simulink model "T_vs_pos_host"  (R2021b)
settings: Solver=ode1  StartTime=0.0  StopTime=inf  FixedStep=1e-3  RelTol=1e-3
libraries: slrealtimeutilitieslib x1, slrealtimeiplib x1
settings Model: Creator=tcraddoc  LastModifiedBy=wasynczu
settings SolverCC: AlgebraicLoopSolver=TrustRegion
settings DataIOCC: ReturnWorkspaceOutputs=off
settings DebuggingCC: SFMachineParentedDataDiag=warning  ArithmeticOperatorsInVariantConditions=warning
settings SFSimCC: SimUseLocalCustomCode=off  CustomCodeUndefinedFunction=UseInterfaceOnly
settings RTWCC: RTWUseLocalCustomCode=off
settings CodeAppCC: StateflowObjectComments=on

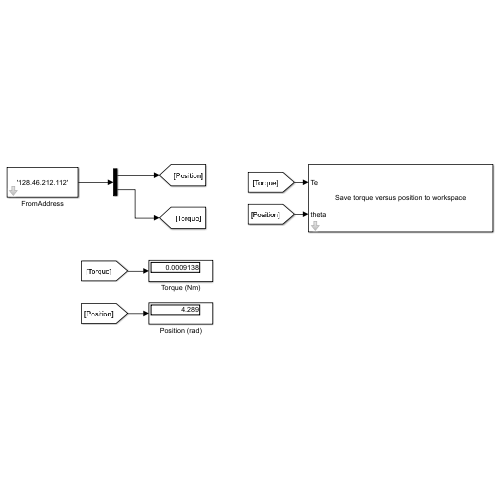
[thumbnail: Simulink's stored preview of the top-level diagram]
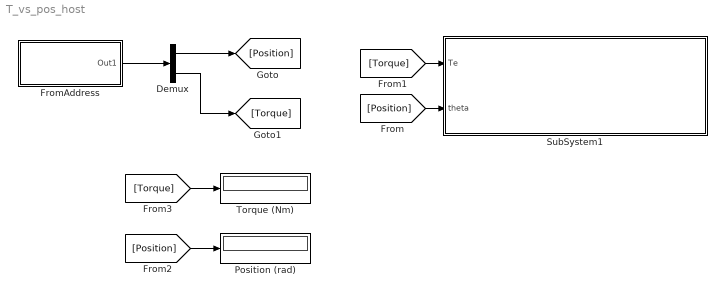
== system T_vs_pos_host ==
  Demux : Demux  Outputs=2
  FromAddress : Subsystem  mask{fromIPAddress='128.46.212.112'}
      mask prompts: fromIPAddress "From IP Address"
      mask Display: disp((get_param(gcb,'fromIPAddress')))
  Position (rad) : Display
  SubSystem1 : Subsystem  mask{N=12}
      mask prompts: N "encoder bits"
      mask help: This block save inductance and position to the Matlab Workspace. The Matlab variables are called "position" and "inductance". The number of encoder bits should be set to that of the encoder you are using (10 in this lab)
      mask init:
      | clear inductance
      | clear position
      | dtheta = 2*pi/(2^N);
      mask Display:
      | disp('Save torque versus position to workspace')
      | port_label('input', 1, 'Te')
      | port_label('input', 2, 'theta')
  Torque (Nm) : Display
  wires:
  Demux/1 -> [Position]
  Demux/2 -> [Torque]
  [Position] -> SubSystem1/2(theta)
  [Torque] -> SubSystem1/1(Te)
  [Torque] -> Torque (Nm)/1
  [Position] -> Position (rad)/1
  FromAddress/1(Out1) -> Demux/1

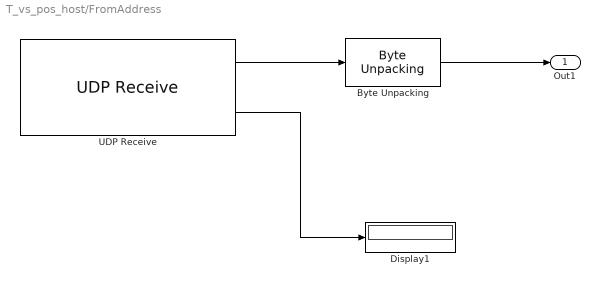
== system T_vs_pos_host/FromAddress ==
  Byte Unpacking : slrealtimeutilitieslib/Byte Unpacking  MaskUnpackedDataTypes={['double']}  MaskUnpackedDataSizes={[2]}  MaskAlignment=1
      settings: SourceProductBaseCode=XP
  Display1 : Display
  UDP Receive : slrealtimeiplib/UDP Receive  useHostTargetConn=on  ipAddress=128.46.212.188  localPort=34  rcvWidth=16  rcvFmAny=off  fmAddress=fromIPAddress  sampleTime=1e-3
      settings: SourceProductBaseCode=XP
  Out1 : Outport
  wires:
  Byte Unpacking/1 -> Out1/1
  UDP Receive/2 -> Display1/1
  UDP Receive/1 -> Byte Unpacking/1

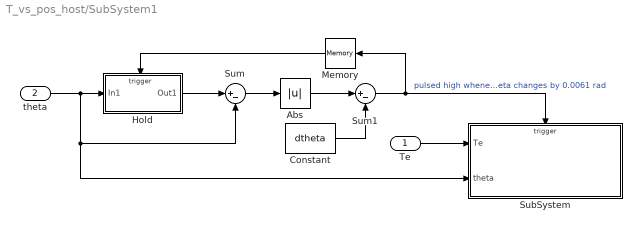
== system T_vs_pos_host/SubSystem1 ==
  Te : Inport
  theta : Inport  Port=2
  Abs : Abs  SaturateOnIntegerOverflow=on
  Constant : Constant  Value=dtheta
  Hold : Subsystem  TreatAsAtomicUnit=on
  Memory : Memory
  SubSystem : Subsystem  TreatAsAtomicUnit=on
  Sum : Sum  Inputs=|+-  InputSameDT=on  SaturateOnIntegerOverflow=on  OutDataTypeStr=Inherit: Same as first input
  Sum1 : Sum  Inputs=|+-  InputSameDT=on  SaturateOnIntegerOverflow=on  OutDataTypeStr=Inherit: Same as first input
  wires:
  Te/1 -> SubSystem/1(Te)
  theta/1 -> Hold/1(In1), Sum/2, SubSystem/2(theta)
  Hold/1(Out1) -> Sum/1
  Sum/1 -> Abs/1
  Abs/1 -> Sum1/1
  Sum1/1 -> SubSystem/Trigger, Memory/1  "pulsed high whenever theta changes by 0.0061 rad"
  Constant/1 -> Sum1/2
  Memory/1 -> Hold/Trigger

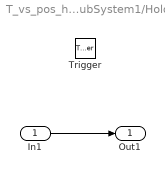
== system T_vs_pos_host/SubSystem1/Hold ==
  In1 : Inport
  Trigger : TriggerPort  VariantControl=Variant
  Out1 : Outport
  wires:
  In1/1 -> Out1/1

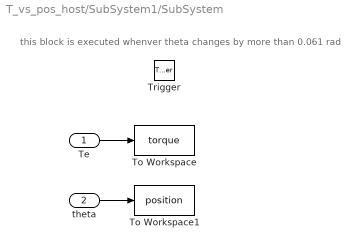
== system T_vs_pos_host/SubSystem1/SubSystem ==
  note: this block is executed whenver theta changes by more than 0.061 rad
  Te : Inport
  theta : Inport  Port=2
  Trigger : TriggerPort  VariantControl=Variant
  To Workspace : ToWorkspace  VariableName=torque  SampleTime=-1
      settings: MaxDataPoints=2^(N+3)
  To Workspace1 : ToWorkspace  VariableName=position  SampleTime=-1
      settings: MaxDataPoints=2^(N+3)
  wires:
  Te/1 -> To Workspace/1
  theta/1 -> To Workspace1/1
